simulink model "PID_controller_tuning"  (R2022a)
settings: Solver=FixedStepAuto  StartTime=0.0  StopTime=inf  RelTol=1e-3
undefined symbols (not defined in the file or in its folder): canChannel
libraries: canlib x3, canmsglib x2, slctrlblks x1, slpidlib x1
settings Model: Creator=Haricharan Projects  LastModifiedBy=Haricharan Projects

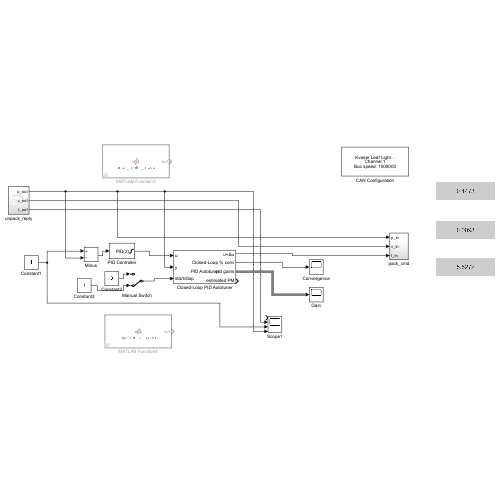
[thumbnail: Simulink's stored preview of the top-level diagram]
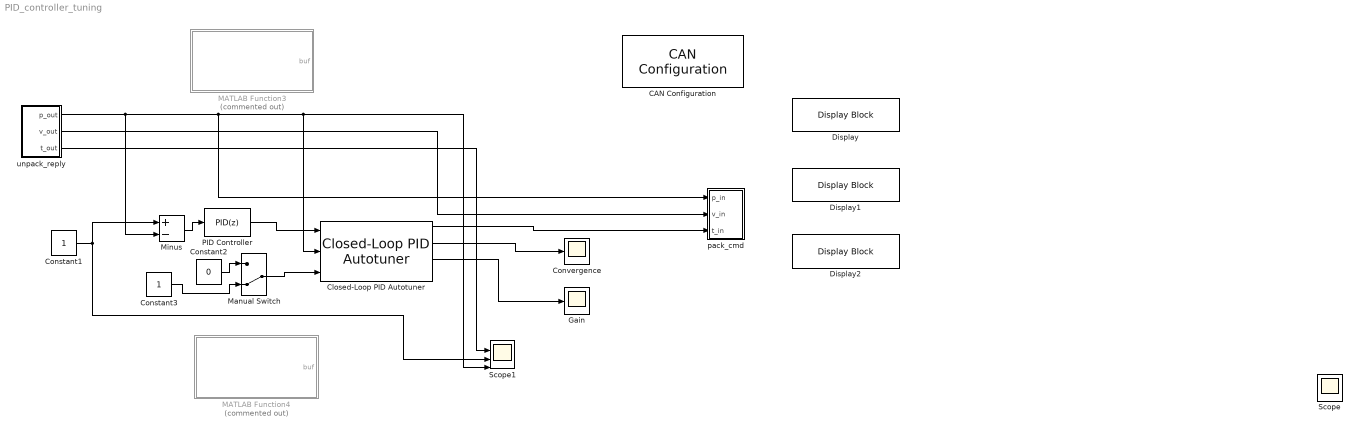
== system PID_controller_tuning ==
  CAN Configuration : canlib/CAN Configuration  BlockHandle=6656.0057  Device=Kvaser Leaf Light v2 1 (Channel 1)  DeviceMenu=Kvaser Leaf Light v2 1 (Channel 1)  ObjConstructor=canChannel('Kvaser', 'Leaf Light v2 1', 1)  BusSpeed=1000000  EnableBitParameters=off  SJW=1  TSEG1=5  TSEG2=2  NSamples=3  AckMode=Normal
      settings: SourceProductBaseCode=VN
  Closed-Loop PID Autotuner : slctrlblks/Closed-Loop PID Autotuner  PIDType=PID  PIDForm=Parallel  TimeDomain=discrete-time  DiscreteTs=0.01  TuningTs=0.2  UseTuningTs=off  IntegratorFormula=Forward Euler  FilterFormula=Forward Euler  ContinuousTs=0.02  Bandwidth=1  UseExternalWC=off  TargetPM=60  UseExternalPM=off  UseExternalAchievedPM=on  ExperimentMode=Superposition  PlantType=Stable  PlantSign=Positive  AmpSine=1  UseExternalAmpSine=off  UseExternalFRD=off  UseExternalU0=off  UseCompanion=off  NotDeployTuningModule=off  UsePLCCoder=off  OutputMode=control action + perturbation  BlockDataType=double  UseConnectedPID=on  blockpath=[]  tunedP=0  tunedI=0  tunedD=0  tunedN=100  tunedPM=0  EstimationWindowSize=3  UseExternalTuningParams=off  OutputChoice=VariantCandD  SingleMultiRateVariant=SingleSamplingRate  ExperimentModeVariant=VariantSuperimposed  NumEstimationPeriods=4  NumSettlingPeriods=2
      settings: SourceProductBaseCode=SD
  Constant1 : Constant
  Constant2 : Constant  Value=0
  Constant3 : Constant
  Convergence : Scope
  Display : DisplayBlock  LabelPosition=Hide  Transparency=1
  Display1 : DisplayBlock  LabelPosition=Hide  Transparency=1
  Display2 : DisplayBlock  LabelPosition=Hide  Transparency=1
  Gain : Scope
  MATLAB Function3 : MATLAB Function  Commented=on  TreatAsAtomicUnit=on
  MATLAB Function4 : MATLAB Function  Commented=on  TreatAsAtomicUnit=on
  Manual Switch : ManualSwitch  CurrentSetting=0
  Minus : Sum  Inputs=+-
  PID Controller : slpidlib/PID Controller  Controller=PID  Form=Parallel  TimeDomain=Discrete-time  UseExternalTs=off  SampleTime=0.01  IntegratorMethod=Forward Euler  FilterMethod=Forward Euler  ControllerParametersSource=internal  P=10  I=0  UseKiTs=off  D=1  N=100  UseFilter=on  TunerSelectOption=Transfer Function Based (PID Tuner App)  InitialConditionSource=internal  InitialConditionForIntegrator=0  InitialConditionForFilter=0  DifferentiatorICPrevScaledInput=0  ExternalReset=none  TrackingMode=off  Kt=1  LimitOutput=on  SatLimitsSource=internal  UpperSaturationLimit=15  LowerSaturationLimit=-15  LinearizeAsGain=on  AntiWindupMode=clamping  Kb=1  POutMin=[]  POutMax=[]  IOutMin=[]  IOutMax=[]  DOutMin=[]  DOutMax=[]  NOutMin=[]  NOutMax=[]  SumOutMin=[]  SumOutMax=[]  SaturationOutMin=[]  SaturationOutMax=[]  PParamMin=[]  PParamMax=[]  IParamMin=[]  IParamMax=[]  DParamMin=[]  DParamMax=[]  NParamMin=[]  NParamMax=[]  KbParamMin=[]  KbParamMax=[]  KtParamMin=[]  KtParamMax=[]  KbOutMin=[]  KbOutMax=[]  KtOutMin=[]  KtOutMax=[]  IntegratorOutMin=[]  IntegratorOutMax=[]  FilterOutMin=[]  FilterOutMax=[]  SumI1OutMin=[]  SumI1OutMax=[]  SumI2OutMin=[]  SumI2OutMax=[]  SumI3OutMin=[]  SumI3OutMax=[]  SumI4OutMin=[]  SumI4OutMax=[]  SumDOutMin=[]  SumDOutMax=[]  DifferentiatorOutMin=[]  DifferentiatorOutMax=[]  FilterDiffOutCoefMin=[]  FilterDiffOutCoefMax=[]  ReciprocalOutMin=[]  ReciprocalOutMax=[]  SumDenOutMin=[]  SumDenOutMax=[]  SumNumOutMin=[]  SumNumOutMax=[]  DivideOutMin=[]  DivideOutMax=[]  UdiffTsProdOutMin=[]  UdiffTsProdOutMax=[]  NTsProdOutMin=[]  NTsProdOutMax=[]  UintegralTsProdOutMin=[]  UintegralTsProdOutMax=[]  UngainTsProdOutMin=[]  UngainTsProdOutMax=[]  IntegratorContinuousStateAttributes=''  IntegratorStateMustResolveToSignalObject=off  IntegratorRTWStateStorageClass=Auto  FilterContinuousStateAttributes=''  FilterStateMustResolveToSignalObject=off  FilterRTWStateStorageClass=Auto  ParallelPVariant=InternalParameters  IdealPVariant=Disabled  IVariant=InternalParameters  DVariant=InternalParameters  IntegratorVariant=Discrete  SatVariant=Enabled  AWVariant=DiscClampingParallel  PCopyVariant=Disabled  TRVariant=Disabled  FdbkBlocksVariant=Forward  IdealPFdbkVariant=Disabled  SatFdbkVariant=Disabled  DerivativeFilterVariant=ForwardEulerFilter  NVariant=InternalParameters  NCopyVariant=Disabled  FilterICVariant=InternalICsFilter  IntegratorICVariant=InternalICs  ExternalResetVariant=Disabled  TRSumVariant=Passthrough  SumFdbkVariant=Disabled  SumVariant=Sum_PID  TsampFilterVariant=InternalTs  TsampNgainVariant=Passthrough  TsampIntegralVariant=Passthrough  ExternalSaturationOutDataTypeStr=Inherit: Same as second input  aMode=0
  Scope1 : Scope  NumInputPorts=4
  pack_cmd : Subsystem
  unpack_reply : Subsystem
  Scope : Scope
  wires:
  unpack_reply/1(p_out) -> Scope1/4, Closed-Loop PID Autotuner/2, pack_cmd/1(p_in), Minus/2
  unpack_reply/2(v_out) -> pack_cmd/2(v_in)
  Constant1/1 -> Scope1/3, Minus/1
  unpack_reply/3(t_out) -> Scope1/2
  Minus/1 -> PID Controller/1
  PID Controller/1 -> Closed-Loop PID Autotuner/1
  Closed-Loop PID Autotuner/1 -> pack_cmd/3(t_in)
  Manual Switch/1 -> Closed-Loop PID Autotuner/3
  Closed-Loop PID Autotuner/3 -> Gain/1
  Closed-Loop PID Autotuner/2 -> Convergence/1
  Constant2/1 -> Manual Switch/1
  Constant3/1 -> Manual Switch/2

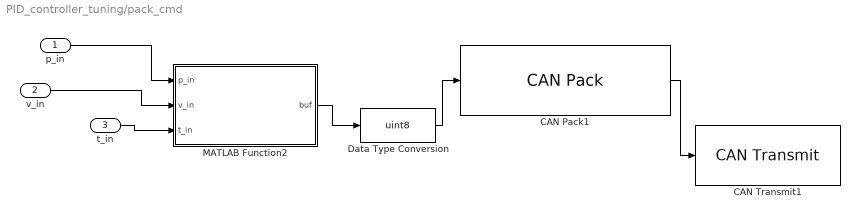
== system PID_controller_tuning/pack_cmd ==
  p_in : Inport
  v_in : Inport  Port=2
  t_in : Inport  Port=3
  CAN Pack1 : canmsglib/CAN Pack  MsgList=(none)  MsgName=CAN Msg  MsgIDType=Standard (11-bit identifier)  MsgIdentifier=1  MsgLength=8  Remote=off  ApplyMinMax=off  BusOutput=off  SignalInfo={}
      settings: SourceProductBaseCode=XP,ME,VN  DataFormat=raw data
  CAN Transmit1 : canlib/CAN Transmit  BlockHandle=6717.0006  Device=Kvaser Leaf Light v2 1 (Channel 1)  DeviceMenu=Kvaser Leaf Light v2 1 (Channel 1)  ObjConstructor=canChannel('Kvaser', 'Leaf Light v2 1', 1)  EnableEventTransmit=off  EnablePeriodicTransmit=on  MessagePeriod=0.01
      settings: SourceProductBaseCode=VN
  Data Type Conversion : DataTypeConversion  OutDataTypeStr=uint8  SaturateOnIntegerOverflow=off  RndMeth=Floor
  MATLAB Function2 : MATLAB Function  TreatAsAtomicUnit=on
  wires:
  CAN Pack1/1 -> CAN Transmit1/1
  MATLAB Function2/1(buf) -> Data Type Conversion/1
  Data Type Conversion/1 -> CAN Pack1/1
  t_in/1 -> MATLAB Function2/3(t_in)
  v_in/1 -> MATLAB Function2/2(v_in)
  p_in/1 -> MATLAB Function2/1(p_in)

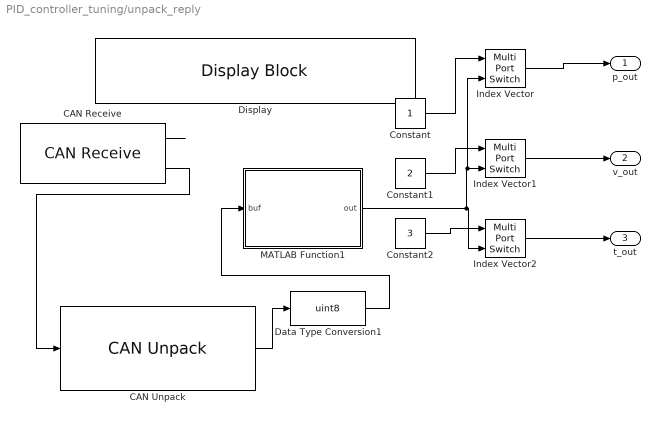
== system PID_controller_tuning/unpack_reply ==
  CAN Receive : canlib/CAN Receive  BlockHandle=6751.0005  Device=Kvaser Leaf Light v2 1 (Channel 1)  DeviceMenu=Kvaser Leaf Light v2 1 (Channel 1)  ObjConstructor=canChannel('Kvaser', 'Leaf Light v2 1', 1)  EnableStandardIDsFilter=off  StdIDsCombo=Allow all  StandardIDs=0  EnableExtendedIDsFilter=off  ExtIDsCombo=Allow all  ExtendedIDs=0  SampleTime=0.01  MsgsPerTimestep=all  InternalFilterUpdateStatus=on  BusOutput=off
      settings: SourceProductBaseCode=VN
  CAN Unpack : canmsglib/CAN Unpack  MsgList=(none)  MsgName=CAN Msg  MsgIDType=Standard (11-bit identifier)  MsgIdentifier=0  MsgLength=8  SignalInfo={}  IDPort=off  TimestampPort=off  ErrorPort=off  RemotePort=off  LengthPort=off  StatusPort=off  ApplyMinMax=off
      settings: SourceProductBaseCode=XP,ME,VN  DataFormat=raw data
  Constant : Constant
  Constant1 : Constant  Value=2
  Constant2 : Constant  Value=3
  Data Type Conversion1 : DataTypeConversion  OutDataTypeStr=uint8  SaturateOnIntegerOverflow=off  RndMeth=Floor
  Display : DisplayBlock  LabelPosition=Bottom  Format=long  Transparency=1
  Index Vector : MultiPortSwitch  Inputs=1  SaturateOnIntegerOverflow=off  InputSameDT=off
  Index Vector1 : MultiPortSwitch  Inputs=1  SaturateOnIntegerOverflow=off  InputSameDT=off
  Index Vector2 : MultiPortSwitch  Inputs=1  SaturateOnIntegerOverflow=off  InputSameDT=off
  MATLAB Function1 : MATLAB Function  TreatAsAtomicUnit=on
  p_out : Outport
  v_out : Outport  Port=2
  t_out : Outport  Port=3
  wires:
  CAN Receive/2 -> CAN Unpack/1
  CAN Receive/1 -> ?
  Data Type Conversion1/1 -> MATLAB Function1/1(buf)
  CAN Unpack/1 -> Data Type Conversion1/1
  Index Vector/1 -> p_out/1
  Index Vector1/1 -> v_out/1
  Index Vector2/1 -> t_out/1
  Constant/1 -> Index Vector/1
  Constant1/1 -> Index Vector1/1
  Constant2/1 -> Index Vector2/1
  MATLAB Function1/1(out) -> Index Vector/2, Index Vector1/2, Index Vector2/2

== matlab function PID_controller_tuning/pack_cmd/MATLAB Function2 ==
  data: p_in input double; buf output; v_in input; t_in input
function buf  = pack_cmd(p_in, v_in, t_in)

P_MIN = -12.5;
P_MAX = 12.5;
V_MIN = -8.0;
V_MAX = 8.0;
KP_MIN = 0.0;
KP_MAX = 500.0;
KD_MIN = 0.0;
KD_MAX = 5.0;
T_MIN = -144.0;
T_MAX = 144.0;

kp_in = 0;
kd_in = 0;

p_des = constrain(p_in, P_MIN, P_MAX);
v_des = constrain(v_in, V_MIN, V_MAX);
kp = constrain(kp_in, KP_MIN, KP_MAX);
kd = constrain(kd_in, KD_MIN, KD_MAX);
t_ff = constrain(t_in, T_MIN, T_MAX);

p_int = float_to_uint(p_des, P_MIN, P_MAX, 16);
v_int = float_to_uint(v_des, V_MIN, V_MAX, 12);
kp_int = float_to_uint(kp, KP_MIN, KP_MAX, 12);
kd_int = float_to_uint(kd, KD_MIN, KD_MAX, 12);
t_int = float_to_uint(t_ff, T_MIN, T_MAX, 12);

buf = ([0 0 0 0 0 0 0 0]);

buf(1) = bitshift(p_int, -8, 'uint64');
buf(2) = bitand(p_int, uint64(0xFF), 'uint64');
buf(3) = bitshift(v_int, -4, 'uint64');
buf(4) = bitor(bitshift(bitand(v_int, uint64(0xF), 'uint64'), +4, 'uint64'), bitshift(kp_int, -8, 'uint64'));
buf(5) = bitand(kp_int, uint64(0xFF), 'uint64');
buf(6) = bitshift(kd_int, -4, 'uint64');
buf(7) = bitor(bitshift(bitand(kd_int, uint64(0xF)), 4, 'uint64'), bitshift(t_int, -8, 'uint64'));
buf(8) = bitand(t_int, uint64(0xFF), 'uint64');

end

function [pgg] = float_to_uint(x, x_min, x_max, bits)
span = x_max - x_min;
offset = x_min;
pgg = uint64(0);

if (bits == 12)
    pgg = (x - offset) * 4095.0/ span;
    pgg = uint64(pgg);
elseif (bits == 16)
    pgg = (x - offset) * 65535.0/ span;
    pgg = uint64(pgg);
pgg = uint64(pgg);
    
end
end

function val = constrain(value, min_value, max_value)
if (value < min_value)
    val = min_value;
elseif (value > max_value)
    val = max_value;
else
    val = value;
end
end

== matlab function PID_controller_tuning/MATLAB Function3 ==
  data: buf output
function buf = enter_motor_mode()

buf = [0 0 0 0 0 0 0 0];

buf(1) = 0xFF;
buf(2) = 0xFF;
buf(3) = 0xFF;
buf(4) = 0xFF;
buf(5) = 0xFF;
buf(6) = 0xFF;
buf(7) = 0xFF;
buf(8) = 0xFC;

end

== matlab function PID_controller_tuning/MATLAB Function4 ==
  data: buf output
function buf = exit_motor_mode()

buf = [0 0 0 0 0 0 0 0];

buf(1) = 0xFF;
buf(2) = 0xFF;
buf(3) = 0xFF;
buf(4) = 0xFF;
buf(5) = 0xFF;
buf(6) = 0xFF;
buf(7) = 0xFF;
buf(8) = 0xFD;

end

== matlab function PID_controller_tuning/unpack_reply/MATLAB Function1 ==
  data: buf input; out output
function out = unpack_reply(buf)

P_MIN = -12.5;
P_MAX = 12.5;
V_MIN = -8.0;
V_MAX = 8.0;
KP_MIN = 0.0;
KP_MAX = 500.0;
KD_MIN = 0.0;
KD_MAX = 5.0;
T_MIN = -144.0;
T_MAX = 144.0;

buf = uint64(buf);

id = buf(1);
p_int = bitor(bitshift(buf(2), 8), buf(3));
v_int = bitor(bitshift(buf(4), 4), bitshift(buf(5), -4));
i_int = bitor(bitshift(bitand(buf(5), uint64(0x0F)), 8), buf(6));

p_out = uint_to_float(p_int, P_MIN, P_MAX, 16);
v_out = uint_to_float(v_int, V_MIN, V_MAX, 12);
t_out = uint_to_float(i_int, -T_MAX, T_MAX, 12);

out = [p_out v_out t_out];

end

function [pgg] = uint_to_float(x_int, x_min, x_max, bits)

span = double(x_max - x_min);
offset = double(x_min);

if (bits == 12)
    pgg = double(x_int) * span / 4095.0 + offset;
elseif (bits == 16)
    pgg = double(x_int) * span / 65535.0 + offset;
end
end
